simulink model "DQ_Power_Flow"  (R2015a)
settings: Solver=ode45  StartTime=0.0  StopTime=inf  RelTol=1e-3
InitFcn:
  | close all;
  | clear all;
  | clc;
libraries: powerlib_extras x6, powerlib_meascontrol x3, simulink x3, powerlib x1
settings Model: Creator=Dr Kashif  LastModifiedBy=Dr Kashif

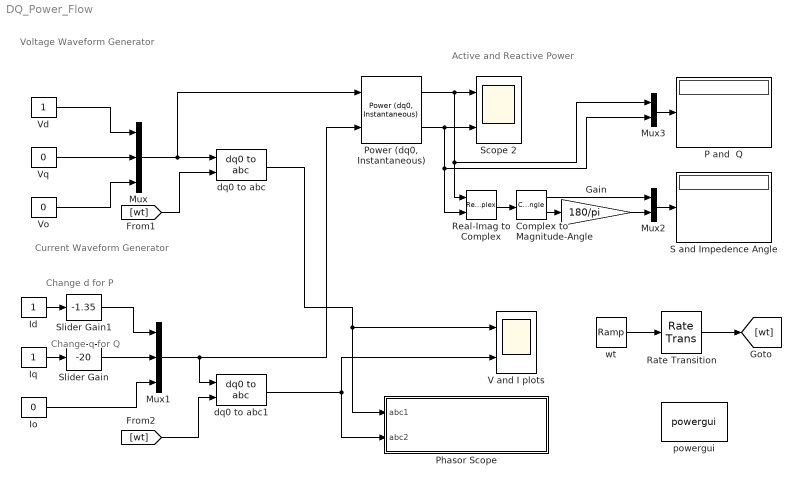
== system DQ_Power_Flow ==
  note: Change q for Q
  note: Change d for P
  note: Active and Reactive Power
  note: Current Waveform Generator
  note: Voltage Waveform Generator
  Complex to Magnitude-Angle : ComplexToMagnitudeAngle
  Gain : Gain  Gain=180/pi
  Id : Constant
  Io : Constant  Value=0
  Iq : Constant
  Mux : Mux  Inputs=3
  Mux1 : Mux  Inputs=3
  Mux2 : Mux  Inputs=2
  Mux3 : Mux  Inputs=2
  P and  Q : Display
  Phasor Scope : Subsystem  mask{f=50, rt=0.5}
      mask prompts: f "Frequency"; rt "Refresh Rate"
      mask Display:
      | port_label('input', 1, 'ABC1')
      | port_label('input', 2, 'ABC2')
  "Power (dq0, Instantaneous)" : powerlib_meascontrol/Measurements/Power (dq0, Instantaneous)
  Rate Transition : RateTransition  OutPortSampleTime=5e-5
  Real-Imag to Complex : RealImagToComplex
  "S and Impedence Angle " : Display
  Scope 2 : Scope  NumInputPorts=2
      settings: TimeRange=0.05  YMin=1.425~1.425  YMax=1.575~1.575
  Slider Gain : simulink/Math Operations/Slider Gain  low=-20  gain=-20  high=20
  Slider Gain1 : simulink/Math Operations/Slider Gain  low=-20  gain=-1.35  high=20
  V and I plots : Scope  NumInputPorts=2
      settings: TimeRange=0.05  YMin=-0.6~-5  YMax=1.2~5
  Vd : Constant
  Vo : Constant  Value=0
  Vq : Constant  Value=0
  dq0 to abc : powerlib_meascontrol/Transformations/dq0 to abc  Alignment=90 degrees behind phase A axis
  dq0 to abc1 : powerlib_meascontrol/Transformations/dq0 to abc  Alignment=90 degrees behind phase A axis
  powergui : powerlib/powergui  Priority=1  SimulationMode=Discrete  SolverType=Tustin/Backward Euler (TBE)  SampleTime=5e-5  frequency=60  SPID=off  DisableSnubberDevices=off  DisableRonSwitches=off  DisableVfSwitches=off  SwTol=0  DisplayEquations=off  Interpol=off  methode=off  Ts=0  FunctionMessages=off  echomessages=off  HookPort=off  EnableUseOfTLC=off  x0status=blocks  frequencyindice=60  Pbase=100e6  ErrMax=1e-4  Iterations=50  UnitsV=kV  UnitsW=MW  buscounter=0  RestoreLinks=warning  ResistiveCurrentMeasurement=off  Frange=[0:2:500]  Ylog=off  Xlog=on  ShowGrid=off  save=off  variable=ZData  structure=0  ZoomFFT=off  StartTime=0.0  cycles=1  DisplayStyle=1  fundamental=60  FreqAxis=off  MaxFrequency=1000  frequencyindicesteady=1  RmsSteady=1  display=off
  wt : simulink/Sources/Ramp  slope=2*pi*50  start=0  X0=0
  wires:
  wt/1 -> Rate Transition/1
  Rate Transition/1 -> [wt]
  [wt] -> dq0 to abc/2
  Vd/1 -> Mux/1
  Vq/1 -> Mux/2
  [wt] -> dq0 to abc1/2
  Mux1/1 -> "Power (dq0, Instantaneous)"/2, dq0 to abc1/1
  Id/1 -> Slider Gain1/1
  Iq/1 -> Slider Gain/1
  Io/1 -> Mux1/3
  "Power (dq0, Instantaneous)"/1 -> Mux3/1, Real-Imag to Complex/1, Scope 2/1
  "Power (dq0, Instantaneous)"/2 -> Mux3/2, Real-Imag to Complex/2, Scope 2/2
  Mux/1 -> "Power (dq0, Instantaneous)"/1, dq0 to abc/1
  Real-Imag to Complex/1 -> Complex to Magnitude-Angle/1
  Complex to Magnitude-Angle/1 -> Mux2/1
  Mux2/1 -> "S and Impedence Angle "/1
  Gain/1 -> Mux2/2
  Complex to Magnitude-Angle/2 -> Gain/1
  dq0 to abc/1 -> Phasor Scope/1(abc1), V and I plots/1
  Vo/1 -> Mux/3
  Slider Gain/1 -> Mux1/2
  dq0 to abc1/1 -> V and I plots/2, Phasor Scope/2(abc2)
  Slider Gain1/1 -> Mux1/1
  Mux3/1 -> P and  Q/1

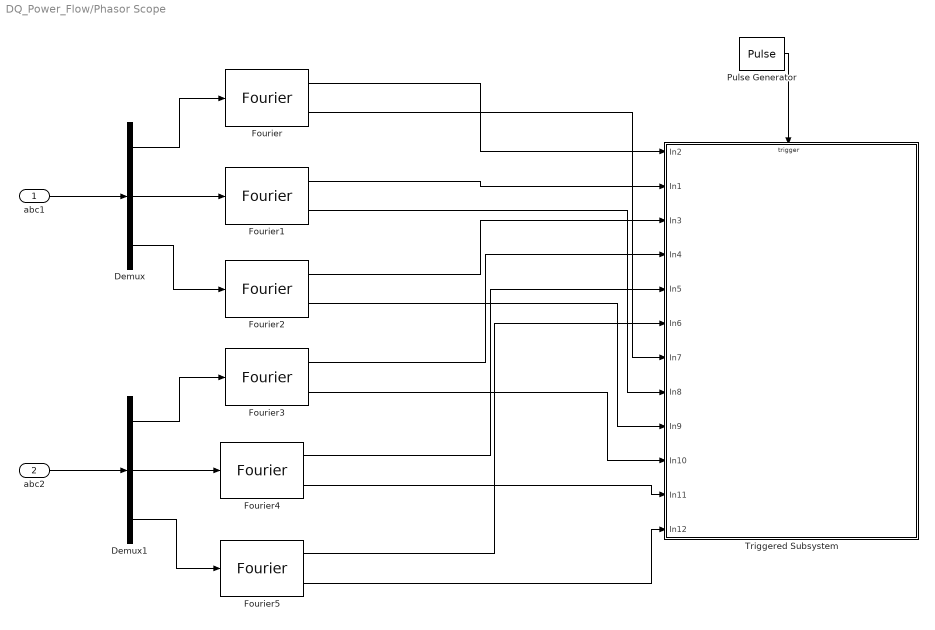
== system DQ_Power_Flow/Phasor Scope ==
  abc1 : Inport
  abc2 : Inport  Port=2
  Demux : Demux  Outputs=3
  Demux1 : Demux  Outputs=3
  Fourier{,1..5} (6 alike) : powerlib_extras/Measurements/Fourier  f1=f  n=1
  Pulse Generator : DiscretePulseGenerator  PulseType=Time based  Period=rt  PulseWidth=10
  Triggered Subsystem : Subsystem  AncestorBlock=|  TreatAsAtomicUnit=on
      | vectorlib/Double System
      | 3-Phase Vector Plotter/Triggered
      | Subsystem
  wires:
  Fourier2/2 -> Triggered Subsystem/9(In9)
  Fourier/1 -> Triggered Subsystem/1(In2)
  Pulse Generator/1 -> Triggered Subsystem/Trigger
  Fourier/2 -> Triggered Subsystem/7(In7)
  Fourier3/2 -> Triggered Subsystem/10(In10)
  Fourier4/2 -> Triggered Subsystem/11(In11)
  Fourier1/1 -> Triggered Subsystem/2(In1)
  Fourier5/1 -> Triggered Subsystem/6(In6)
  Fourier3/1 -> Triggered Subsystem/4(In4)
  Fourier2/1 -> Triggered Subsystem/3(In3)
  Fourier4/1 -> Triggered Subsystem/5(In5)
  Fourier1/2 -> Triggered Subsystem/8(In8)
  Fourier5/2 -> Triggered Subsystem/12(In12)
  Demux/1 -> Fourier/1
  Demux/2 -> Fourier1/1
  Demux/3 -> Fourier2/1
  abc1/1 -> Demux/1
  Demux1/1 -> Fourier3/1
  Demux1/2 -> Fourier4/1
  Demux1/3 -> Fourier5/1
  abc2/1 -> Demux1/1

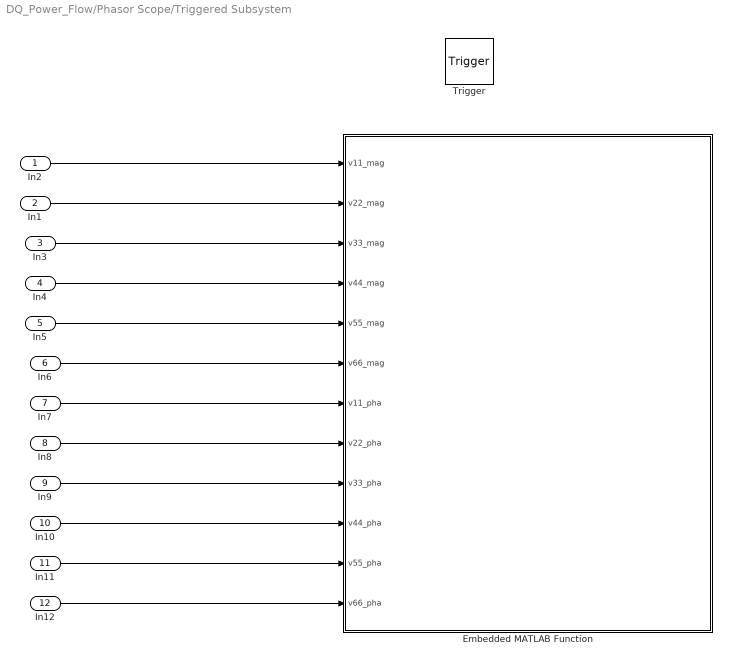
== system DQ_Power_Flow/Phasor Scope/Triggered Subsystem ==
  In2 : Inport
  In1 : Inport  Port=2
  In3 : Inport  Port=3
  In4 : Inport  Port=4
  In5 : Inport  Port=5
  In6 : Inport  Port=6
  In7 : Inport  Port=7
  In8 : Inport  Port=8
  In9 : Inport  Port=9
  In10 : Inport  Port=10
  In11 : Inport  Port=11
  In12 : Inport  Port=12
  Trigger : TriggerPort
  Embedded MATLAB Function : MATLAB Function  TreatAsAtomicUnit=on
  wires:
  In2/1 -> Embedded MATLAB Function/1(v11_mag)
  In1/1 -> Embedded MATLAB Function/2(v22_mag)
  In3/1 -> Embedded MATLAB Function/3(v33_mag)
  In4/1 -> Embedded MATLAB Function/4(v44_mag)
  In5/1 -> Embedded MATLAB Function/5(v55_mag)
  In6/1 -> Embedded MATLAB Function/6(v66_mag)
  In7/1 -> Embedded MATLAB Function/7(v11_pha)
  In8/1 -> Embedded MATLAB Function/8(v22_pha)
  In9/1 -> Embedded MATLAB Function/9(v33_pha)
  In10/1 -> Embedded MATLAB Function/10(v44_pha)
  In11/1 -> Embedded MATLAB Function/11(v55_pha)
  In12/1 -> Embedded MATLAB Function/12(v66_pha)

== matlab function DQ_Power_Flow/Phasor Scope/Triggered Subsystem/Embedded MATLAB Function ==
  data: v11_mag input; v22_mag input; v33_mag input; v44_mag input; v55_mag input; v66_mag input; v11_pha input; v22_pha input; v33_pha input; v44_pha input; v55_pha input; v66_pha input
%-------------------------------------------------------------------------------------------------------------
% Dr. Syed Abdul Rahman Kashif
% Department of Electrical Engineering
% UET, Lahore
%-------------------------------------------------------------------------------------------------------------

function Vector_Diagram_Plotter(v11_mag,v22_mag,v33_mag,v44_mag,v55_mag,v66_mag,v11_pha,v22_pha,v33_pha,v44_pha,v55_pha,v66_pha)

%-------------------------------------------------------------------------------------------------------------

%set(gcf,'DockControl','off')
%set(gcf,'MenuBar','none')

%-------------------------------------------------------------------------------------------------------------
figure(3)
subplot(1,2,1)
polar([0 (v11_pha)*pi/180 0 (v22_pha)*pi/180 0 (v33_pha)*pi/180],[0 v11_mag 0 v22_mag 0 v33_mag]);
grid on;
title(['Voltage Phasors'])

x1=v11_mag*cosd(v11_pha);
y1=v11_mag*sind(v11_pha);

x2=v22_mag*cosd(v22_pha);
y2=v22_mag*sind(v22_pha);

x3=v33_mag*cosd(v33_pha);
y3=v33_mag*sind(v33_pha);

text(x1,y1,'A1')
text(x2,y2,'B1')
text(x3,y3,'C1')

%---------------------------------------------
subplot(1,2,2)
polar([0 (v44_pha)*pi/180 0 (v55_pha)*pi/180 0 (v66_pha)*pi/180],[0 v44_mag 0 v55_mag 0 v66_mag],'r');
grid on;
title('Current Phasors')
%-------------------------------------------------------------------------------------------------------------

x4=v44_mag*cosd(v44_pha);
y4=v44_mag*sind(v44_pha);

x5=v55_mag*cosd(v55_pha);
y5=v55_mag*sind(v55_pha);

x6=v66_mag*cosd(v66_pha);
y6=v66_mag*sind(v66_pha);

text(x4,y4,'A2')
text(x5,y5,'B2')
text(x6,y6,'C2')


%--------------------------------------------------------------------------------------------------------------
